simulink model "freq_response_pendulum"  (R2025b)
settings: Solver=ode45  StartTime=0.0  StopTime=2  RelTol=1e-3
settings Model: Creator=fred  LastModifiedBy=fred

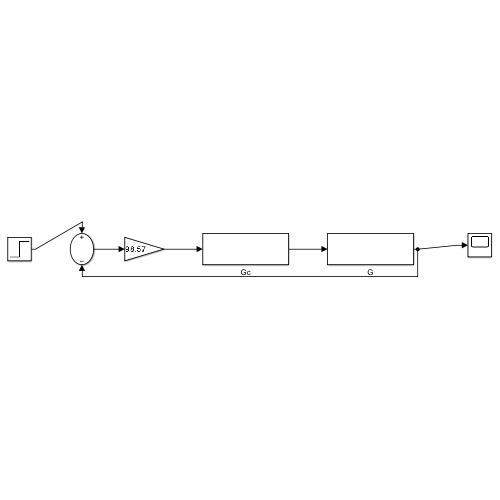
[thumbnail: Simulink's stored preview of the top-level diagram]
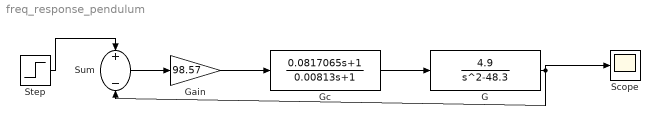
== system freq_response_pendulum ==
  G : TransferFcn  Numerator=[4.9]  Denominator=[1 0 -48.3]
  Gain : Gain  Gain=98.57
  Gc : TransferFcn  Numerator=[0.0817065 1]  Denominator=[0.00813 1]
  Scope : Scope
  Step : Step  SampleTime=0
  Sum : Sum  Inputs=+-
  wires:
  Step/1 -> Sum/1
  Sum/1 -> Gain/1
  Gain/1 -> Gc/1
  Gc/1 -> G/1
  G/1 -> Scope/1, Sum/2
